simulink model "specWindowSHGC"  (R2018b)
settings: Solver=ode45  StartTime=0  StopTime=3600  MaxStep=600  RelTol=1e-3  EnableMultiTasking=on
libraries: carnot x6
settings Model: Creator=drhf  LastModifiedBy=drhf
settings DataIOCC: LimitDataPoints=on  SaveFormat=Array
settings OptimizationCC: DefaultParameterBehavior=Inlined  LifeSpan=inf
settings DebuggingCC: UnderspecifiedInitializationDetection=Classic  MergeDetectMultiDrivingBlocksExec=none  SolverPrmCheckMsg=warning  SFUnexpectedBacktrackingDiag=warning  SFNoUnconditionalDefaultTransitionDiag=warning  SFExecutionAtInitializationDiag=none
settings HardwareCC: ProdBitPerPointer=32  ProdBitPerSizeT=32  ProdBitPerPtrDiffT=32  ProdLargestAtomicFloat=None  ProdIntDivRoundTo=Undefined  ProdEndianess=Unspecified  ProdWordSize=32  ProdHWDeviceType=32-bit Generic
settings ModelReferenceCC: PropagateSignalLabelsOutOfModel=off
settings SFSimCC: SimUseLocalCustomCode=off
settings RTWCC: RTWUseLocalCustomCode=off
settings CodeAppCC: StateflowObjectComments=on
settings GRTTargetCC: TargetLangStandard=C89/C90 (ANSI)  GeneratePreprocessorConditionals=Disable all
settings ConfigComp: CovMetricSettings=dw  CovHtmlReporting=on  CovSaveCumulativeToWorkspaceVar=on  CovSaveSingleToWorkspaceVar=on  CovExternalEMLEnable=off

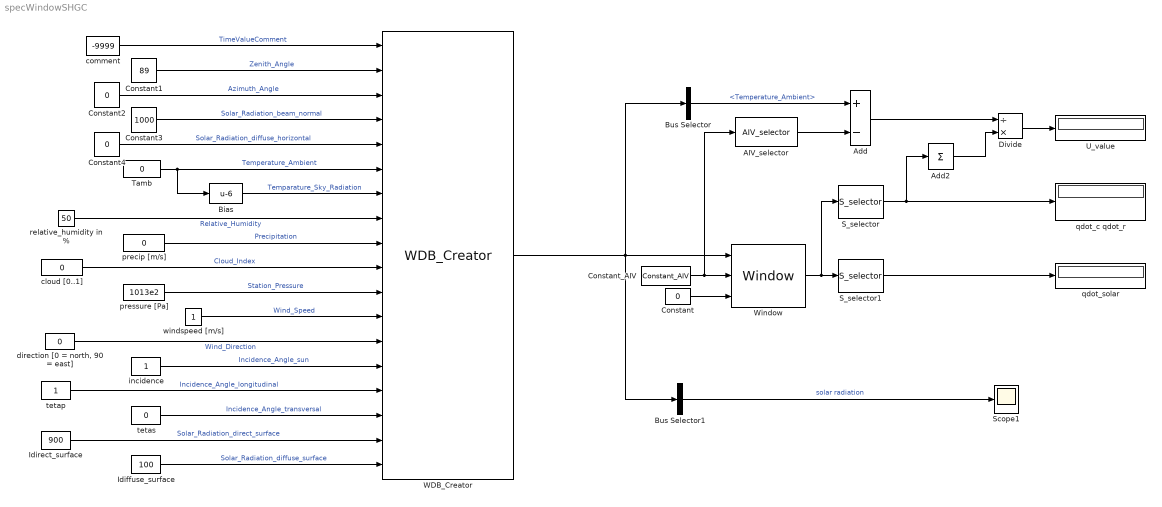
== system specWindowSHGC ==
  AIV_selector : carnot/Outputs/AIV_selector  e1=on  e2=off  e3=off  e4=off  e5=off  e6=off  e7=off  e8=off  e9=off
      settings: SourceProductName=Carnot
  Add : Sum  Inputs=+-
  Add2 : Sum  Inputs=1
  Bias : Bias  Bias=-6
  Bus Selector : BusSelector  OutputSignals=Temperature_Ambient
  Bus Selector1 : BusSelector  OutputSignals=Solar_Radiation_direct_surface,Solar_Radiation_diffuse_surface  OutputAsBus=on
  Constant : Constant  Value=0
  Constant1 : Constant  Value=89
  Constant2 : Constant  Value=0
  Constant3 : Constant  Value=1000
  Constant4 : Constant  Value=0
  Constant_AIV : carnot/Source/Ventilation/Constant_AIV  Tsens=20  Tcon=20  Trad=20  mw=0.012  mco=0.01  rhoair=1.2  cpair=1004  pair=100000  nair=0.5
      settings: SourceProductName=Carnot
  Divide : Product  Inputs=/*
  Idiffuse_surface : Constant  Value=100
  Idirect_surface : Constant  Value=900
  S_selector : carnot/Outputs/S_selector  e1=off  e2=off  e3=off  e4=off  e5=off  e6=off  e7=on  e8=on  e9=off  e10=off  e11=off  e12=off  e13=off
      settings: SourceProductName=Carnot
  S_selector1 : carnot/Outputs/S_selector  e1=on  e2=off  e3=off  e4=off  e5=off  e6=off  e7=off  e8=off  e9=off  e10=off  e11=off  e12=off  e13=off
      settings: SourceProductName=Carnot
  Scope1 : Scope
  Tamb : Constant  Value=0
  U_value : Display
  WDB_Creator : carnot/Basic/Weather_and_Sun/WDB_Creator
      settings: SourceProductName=Carnot
  Window : carnot/Basic/Thermal_Models/Window  pos=0  windowsize=[1 1]  frame=0  Ug=1.8  gvalue=0.6  tauzero=0.6  numpanes=2  d=[0.004 0.004]  rho=[2500 2500]  cp="[1008  1008]"  t0=20  misc=[0.2 0.1 1 1]  shad_type=No shading  type_glazing=double glazing normal  tau_shad=0.01  bli_a=0.05  bli_b=1  bli_c=0.05  bli_d=0.05  bli_alpha=90  bli_refl=0.2
      settings: SourceProductName=Carnot
  cloud [0..1] : Constant  Value=0
  comment : Constant  Value=-9999
  "direction [0 = north, 90 = east]" : Constant  Value=0
  incidence : Constant
  precip [m/s] : Constant  Value=0
  pressure [Pa] : Constant  Value=1013e2
  qdot_c qdot_r : Display
  qdot_solar : Display
  relative_humidity in % : Constant  Value=50
  tetap : Constant
  tetas : Constant  Value=0
  windspeed [m/s] : Constant
  wires:
  WDB_Creator/1 -> Window/1, Bus Selector/1, Bus Selector1/1
  Constant_AIV/1 -> Window/2, AIV_selector/1
  Window/1 -> S_selector1/1, S_selector/1
  S_selector/1 -> Add2/1, qdot_c qdot_r/1
  AIV_selector/1 -> Add/2
  Add/1 -> Divide/1
  Add2/1 -> Divide/2
  Divide/1 -> U_value/1
  Constant/1 -> Window/3
  Bus Selector/1 -> Add/1  "<Temperature_Ambient>"
  Bus Selector1/1 -> Scope1/1  "solar radiation"
  incidence/1 -> WDB_Creator/14  "Incidence_Angle_sun"
  "direction [0 = north, 90 = east]"/1 -> WDB_Creator/13  "Wind_Direction"
  tetap/1 -> WDB_Creator/15  "Incidence_Angle_longitudinal"
  Idiffuse_surface/1 -> WDB_Creator/18  "Solar_Radiation_diffuse_surface"
  pressure [Pa]/1 -> WDB_Creator/11  "Station_Pressure"
  Bias/1 -> WDB_Creator/7  "Temparature_Sky_Radiation"
  Constant2/1 -> WDB_Creator/3  "Azimuth_Angle"
  Constant1/1 -> WDB_Creator/2  "Zenith_Angle"
  Constant4/1 -> WDB_Creator/5  "Solar_Radiation_diffuse_horizontal"
  precip [m/s]/1 -> WDB_Creator/9  "Precipitation"
  cloud [0..1]/1 -> WDB_Creator/10  "Cloud_Index"
  comment/1 -> WDB_Creator/1  "TimeValueComment"
  Idirect_surface/1 -> WDB_Creator/17  "Solar_Radiation_direct_surface"
  relative_humidity in %/1 -> WDB_Creator/8  "Relative_Humidity"
  Tamb/1 -> WDB_Creator/6, Bias/1  "Temperature_Ambient"
  Constant3/1 -> WDB_Creator/4  "Solar_Radiation_beam_normal"
  windspeed [m/s]/1 -> WDB_Creator/12  "Wind_Speed"
  tetas/1 -> WDB_Creator/16  "Incidence_Angle_transversal"
  S_selector1/1 -> qdot_solar/1
